simulink library "tp333079"  (Simulink 5.0)
values from neighbouring files (symbols this model uses):
  b = 1    [main_flock3.m]    (also in main_flock4.m; params_flocking_ros.m)
undefined symbols (not defined in the file or in its folder): AC, AlphaBnd, BetaBnd, CDda, CDde, CDdf, CDdr, CDM, CDmin, CGempty, CGgross, CL0, CLa, CLalphadot, Clbeta, Clda, CLde, CLdf, Cldr, CLM, CLmind, Clp, CLq, Clr, Cm0, Cma, Cmalphadot, Cmde, Cmdf, CmM, Cmq, Cnbeta, Cnda, Cndr, Cnp, Cnr, CP, CT, CYbeta, CYda, CYdr, CYp, CYr, Displacement, dmy, Engine, EulerIni, FuelFlow, FuelIni, J, Jempty, Jeng, Jgross, Jprop, MAC, MAP, MAPLim, MassIni, MaxPower, mempty ... (+26)
libraries: aerosimlib x325, simulink3 x42
(part 6 of 11)

== system tp333079/Complete Aircraft/6-DOF Aircraft Model (Body-frame EOM)/Atmosphere ==
  note: Inputs
  note: Outputs
  MSL : Inport  Port=1  PortDimensions=1  SampleTime=-1  DataType=double
      settings: SignalType=auto
  AGL : Inport  Port=2  PortDimensions=1  SampleTime=-1  DataType=double
      settings: SignalType=auto
  Winds : Inport  Port=3  PortDimensions=[3 1]  SampleTime=-1  DataType=double
      settings: SignalType=auto
  VelB : Inport  Port=4  PortDimensions=[3 1]  SampleTime=-1  DataType=double
      settings: SignalType=auto
  VelW : Inport  Port=5  PortDimensions=[3 1]  SampleTime=-1  DataType=auto
      settings: SignalType=auto
  DCM : Inport  Port=6  PortDimensions=[3 3]  SampleTime=-1  DataType=double
      settings: SignalType=auto
  Background Wind : aerosimlib/Atmosphere/Background Wind
  Standard Atmosphere : aerosimlib/Atmosphere/Standard Atmosphere
  Sum : Sum  Inputs=|++  SaturateOnIntegerOverflow=on
  Turbulence : aerosimlib/Atmosphere/Turbulence  tsamp=tsamp
  Wind Shear : aerosimlib/Atmosphere/Wind Shear
  pstatic : Outport  Port=1
  OAT : Outport  Port=2
  rho : Outport  Port=3
  a : Outport  Port=4
  WindVel : Outport  Port=5
  WindRates : Outport  Port=6
  wires:
  MSL/1 -> Standard Atmosphere/1
  Winds/1 -> Background Wind/1
  DCM/1 -> Background Wind/2
  Background Wind/1 -> Turbulence/3, Sum/2
  AGL/1 -> Turbulence/2
  VelW/1 -> Turbulence/1
  Background Wind/2 -> Wind Shear/1
  Turbulence/1 -> Sum/1
  Turbulence/2 -> Wind Shear/2
  VelB/1 -> Wind Shear/3
  Wind Shear/1 -> WindRates/1
  Standard Atmosphere/1 -> pstatic/1
  Standard Atmosphere/2 -> OAT/1
  Standard Atmosphere/3 -> rho/1
  Standard Atmosphere/4 -> a/1
  Sum/1 -> WindVel/1

== system tp333079/Complete Aircraft/6-DOF Aircraft Model (Body-frame EOM)/Earth ==
  note: Inputs
  note: Outputs
  Position : Inport  Port=1  PortDimensions=[3 1]  SampleTime=-1  DataType=double
      settings: SignalType=auto
  DCM : Inport  Port=2  PortDimensions=[3 3]  SampleTime=-1  DataType=double
      settings: SignalType=auto
  Demux : Demux  Outputs=2  BusSelectionMode=off
  ECEF Position : aerosimlib/Transformations/ECEF Position
  EGM-96 : aerosimlib/Earth/EGM-96
  Ground Alt : Constant  Value=GndAlt
  Ground Detection : aerosimlib/Earth/Ground Detection
  Mux3 : Mux  Inputs=2
  WGS-84 : aerosimlib/Earth/WGS-84
  WMM-2000 : aerosimlib/Earth/WMM-2000  wmmfile=wmmfile  simdate=dmy
  MSL : Outport  Port=1
  AGL : Outport  Port=2
  AConGnd : Outport  Port=3
  Rearth : Outport  Port=4
  Requiv : Outport  Port=5
  Gravity : Outport  Port=6
  MagField : Outport  Port=7
  ECEF : Outport  Port=8
  wires:
  Position/1 -> WGS-84/1, EGM-96/1, WMM-2000/1, ECEF Position/1
  DCM/1 -> WMM-2000/2
  Ground Alt/1 -> Ground Detection/2
  EGM-96/1 -> Ground Detection/1, MSL/1
  WGS-84/1 -> Mux3/1
  WGS-84/2 -> Mux3/2
  Ground Detection/2 -> AGL/1
  Ground Detection/1 -> AConGnd/1
  Mux3/1 -> Rearth/1, Demux/1
  WGS-84/3 -> Requiv/1
  WGS-84/4 -> Gravity/1
  WMM-2000/1 -> MagField/1
  Demux/1 -> ECEF Position/2
  Demux/2 -> ECEF Position/3
  ECEF Position/1 -> ECEF/1

== system tp333079/Complete Aircraft/6-DOF Aircraft Model (Body-frame EOM)/Equations of Motion ==
  note: Outputs
  note: Inputs
  Accel : Inport  Port=1  PortDimensions=[3 1]  SampleTime=-1  DataType=auto
      settings: SignalType=auto
  Moment : Inport  Port=2  PortDimensions=[3 1]  SampleTime=-1  DataType=auto
      settings: SignalType=auto
  Inertia : Inport  Port=3  PortDimensions=[4 1]  SampleTime=-1  DataType=auto
      settings: SignalType=auto
  Rearth : Inport  Port=4  PortDimensions=[2 1]  SampleTime=-1  DataType=auto
      settings: SignalType=auto
  Gravity : Inport  Port=5  PortDimensions=1  SampleTime=-1  DataType=auto
      settings: SignalType=auto
  AConGnd : Inport  Port=6  PortDimensions=1  SampleTime=-1  DataType=auto
      settings: SignalType=auto
  RST : Inport  Port=7  PortDimensions=1  SampleTime=-1  DataType=auto
      settings: SignalType=auto
  Body-Inertial DCM From Quaternions : aerosimlib/Transformations/Body-Inertial DCM From Quaternions
  Demux : Demux  Outputs=2  BusSelectionMode=off
  Euler Angles From Quaternions : aerosimlib/Transformations/Euler Angles From Quaternions
  Forces : aerosimlib/Equations of Motion/Body-Frame EOM/Forces  VelocitiesIni=VelocitiesIni
  Kinematics (Quaternions) : aerosimlib/Equations of Motion/Body-Frame EOM/Kinematics (Quaternions)  QuaternionsIni=QuaternionsIni
  Moments : aerosimlib/Equations of Motion/Body-Frame EOM/Moments  RatesIni=RatesIni
  Navigation : aerosimlib/Equations of Motion/Body-Frame EOM/Navigation  PositionIni=PositionIni
  VelB : Outport  Port=1
  Rates : Outport  Port=2
  Quaternions : Outport  Port=3
  Position : Outport  Port=4
  Groundspeed : Outport  Port=5
  DCM : Outport  Port=6
  Euler : Outport  Port=7
  Ang Acc : Outport  Port=8
  wires:
  Euler Angles From Quaternions/1 -> Euler/1
  Body-Inertial DCM From Quaternions/1 -> DCM/1, Forces/4, Navigation/2
  Rearth/1 -> Demux/1
  Demux/1 -> Navigation/3
  Demux/2 -> Navigation/4
  Accel/1 -> Forces/2
  Moment/1 -> Moments/2
  Inertia/1 -> Moments/1
  Gravity/1 -> Forces/3
  AConGnd/1 -> Navigation/5
  Forces/1 -> VelB/1, Navigation/1
  Kinematics (Quaternions)/1 -> Quaternions/1, Euler Angles From Quaternions/1, Body-Inertial DCM From Quaternions/1
  Moments/1 -> Forces/1, Kinematics (Quaternions)/1, Rates/1
  RST/1 -> Forces/5, Moments/3, Navigation/6, Kinematics (Quaternions)/2
  Moments/2 -> Ang Acc/1
  Navigation/1 -> Position/1
  Navigation/2 -> Groundspeed/1

== system tp333079/Complete Aircraft/6-DOF Aircraft Model (Geodetic-frame EOM)/Aerodynamics ==
  note: Aerodynamic Loads
  note: Aerodynamic Coefficients
  note: Aerodynamic Parameters
  note: Outputs
  note: Inputs
  VelB : Inport  Port=1  PortDimensions=[3 1]  SampleTime=-1  DataType=auto
      settings: SignalType=auto
  WindB : Inport  Port=2  PortDimensions=[3 1]  SampleTime=-1  DataType=auto
      settings: SignalType=auto
  Rates : Inport  Port=3  PortDimensions=[3 1]  SampleTime=-1  DataType=auto
      settings: SignalType=auto
  WindRates : Inport  Port=4  PortDimensions=[3 1]  SampleTime=-1  DataType=auto
      settings: SignalType=auto
  AeroCon : Inport  Port=5  PortDimensions=[4 1]  SampleTime=-1  DataType=auto
      settings: SignalType=auto
  rho : Inport  Port=6  PortDimensions=1  SampleTime=-1  DataType=auto
      settings: SignalType=auto
  a : Inport  Port=7  PortDimensions=1  SampleTime=-1  DataType=auto
      settings: SignalType=auto
  Aerodynamic Force : aerosimlib/Aerodynamics/Aerodynamic Force  S=S
  Aerodynamic Moment : aerosimlib/Aerodynamics/Aerodynamic Moment  c=MAC  b=b  S=S
  Drag Coefficient : aerosimlib/Aerodynamics/Drag Coefficient  CL0=CLmind  CD0=CDmin  CDdf=CDdf  CDde=CDde  CDda=CDda  CDdr=CDdr  CDM=CDM  e=osw  b=b  S=S
  Dynamic Pressure : aerosimlib/Aerodynamics/Dynamic Pressure
  Lift Coefficient : aerosimlib/Aerodynamics/Lift Coefficient  CL0=CL0  CLalpha=CLa  CLdf=CLdf  CLde=CLde  CLalphadot=CLalphadot  CLq=CLq  CLM=CLM  c=MAC
  Mux : Mux  Inputs=6
  Pitch Moment Coefficient : aerosimlib/Aerodynamics/Pitch Moment Coefficient  Cm0=Cm0  Cma=Cma  Cmdf=Cmdf  Cmde=Cmde  Cmalphadot=Cmalphadot  Cmq=Cmq  CmM=CmM  c=MAC
  Roll Moment Coefficient : aerosimlib/Aerodynamics/Roll Moment Coefficient  Clbeta=Clbeta  Clda=Clda  Cldr=Cldr  Clp=Clp  Clr=Clr  b=b
  Side Force Coefficient : aerosimlib/Aerodynamics/Side Force Coefficient  CYbeta=CYbeta  CYda=CYda  CYdr=CYdr  CYp=CYp  CYr=CYr  b=b
  Sum : Sum  Inputs=|+-  SaturateOnIntegerOverflow=on
  Wind-axes Velocities : aerosimlib/Aerodynamics/Wind-axes Velocities  Vabnd=VaBnd  betabnd=BetaBnd  alphabnd=AlphaBnd
  Yaw Moment Coefficient : aerosimlib/Aerodynamics/Yaw Moment Coefficient  Cnbeta=Cnbeta  Cnda=Cnda  Cndr=Cndr  Cnp=Cnp  Cnr=Cnr  b=b
  Faero : Outport  Port=1
  Maero : Outport  Port=2
  AeroCoeff : Outport  Port=3
  VelW : Outport  Port=4
  Mach : Outport  Port=5
  pdyn : Outport  Port=6
  wires:
  VelB/1 -> Wind-axes Velocities/1
  WindB/1 -> Wind-axes Velocities/2
  a/1 -> Wind-axes Velocities/3
  Wind-axes Velocities/1 -> Lift Coefficient/1, Dynamic Pressure/1, Drag Coefficient/1, Side Force Coefficient/1, Pitch Moment Coefficient/1, Roll Moment Coefficient/1, Yaw Moment Coefficient/1, Aerodynamic Force/5, VelW/1
  rho/1 -> Dynamic Pressure/2
  AeroCon/1 -> Lift Coefficient/2, Drag Coefficient/2, Side Force Coefficient/2, Pitch Moment Coefficient/2, Roll Moment Coefficient/2, Yaw Moment Coefficient/2
  Wind-axes Velocities/2 -> Lift Coefficient/3, Pitch Moment Coefficient/3
  Wind-axes Velocities/3 -> Drag Coefficient/4, Pitch Moment Coefficient/5, Lift Coefficient/5, Mach/1
  Lift Coefficient/1 -> Aerodynamic Force/3, Drag Coefficient/3, Mux/3
  Drag Coefficient/1 -> Aerodynamic Force/1, Mux/1
  Side Force Coefficient/1 -> Aerodynamic Force/2, Mux/2
  Dynamic Pressure/1 -> Aerodynamic Force/4, Aerodynamic Moment/4, pdyn/1
  Roll Moment Coefficient/1 -> Aerodynamic Moment/1, Mux/4
  Pitch Moment Coefficient/1 -> Aerodynamic Moment/2, Mux/5
  Yaw Moment Coefficient/1 -> Aerodynamic Moment/3, Mux/6
  Aerodynamic Force/1 -> Faero/1
  Aerodynamic Moment/1 -> Maero/1
  Mux/1 -> AeroCoeff/1
  Rates/1 -> Sum/1
  WindRates/1 -> Sum/2
  Sum/1 -> Lift Coefficient/4, Side Force Coefficient/3, Pitch Moment Coefficient/4, Yaw Moment Coefficient/3, Roll Moment Coefficient/3

== system tp333079/Complete Aircraft/6-DOF Aircraft Model (Geodetic-frame EOM)/Atmosphere ==
  note: Inputs
  note: Outputs
  MSL : Inport  Port=1  PortDimensions=1  SampleTime=-1  DataType=double
      settings: SignalType=auto
  AGL : Inport  Port=2  PortDimensions=1  SampleTime=-1  DataType=double
      settings: SignalType=auto
  Winds : Inport  Port=3  PortDimensions=[3 1]  SampleTime=-1  DataType=double
      settings: SignalType=auto
  VelB : Inport  Port=4  PortDimensions=[3 1]  SampleTime=-1  DataType=double
      settings: SignalType=auto
  VelW : Inport  Port=5  PortDimensions=[3 1]  SampleTime=-1  DataType=auto
      settings: SignalType=auto
  DCM : Inport  Port=6  PortDimensions=[3 3]  SampleTime=-1  DataType=double
      settings: SignalType=auto
  Background Wind : aerosimlib/Atmosphere/Background Wind
  Standard Atmosphere : aerosimlib/Atmosphere/Standard Atmosphere
  Sum : Sum  Inputs=|++  SaturateOnIntegerOverflow=on
  Turbulence : aerosimlib/Atmosphere/Turbulence  tsamp=tsamp
  Wind Shear : aerosimlib/Atmosphere/Wind Shear
  pstatic : Outport  Port=1
  OAT : Outport  Port=2
  rho : Outport  Port=3
  a : Outport  Port=4
  WindVel : Outport  Port=5
  WindRates : Outport  Port=6
  wires:
  MSL/1 -> Standard Atmosphere/1
  Winds/1 -> Background Wind/1
  DCM/1 -> Background Wind/2
  Background Wind/1 -> Turbulence/3, Sum/2
  AGL/1 -> Turbulence/2
  VelW/1 -> Turbulence/1
  Background Wind/2 -> Wind Shear/1
  Turbulence/1 -> Sum/1
  Turbulence/2 -> Wind Shear/2
  VelB/1 -> Wind Shear/3
  Wind Shear/1 -> WindRates/1
  Standard Atmosphere/1 -> pstatic/1
  Standard Atmosphere/2 -> OAT/1
  Standard Atmosphere/3 -> rho/1
  Standard Atmosphere/4 -> a/1
  Sum/1 -> WindVel/1

== system tp333079/Complete Aircraft/6-DOF Aircraft Model (Geodetic-frame EOM)/Earth ==
  note: Inputs
  note: Outputs
  Position : Inport  Port=1  PortDimensions=[3 1]  SampleTime=-1  DataType=double
      settings: SignalType=auto
  DCM : Inport  Port=2  PortDimensions=[3 3]  SampleTime=-1  DataType=double
      settings: SignalType=auto
  Demux : Demux  Outputs=2  BusSelectionMode=off
  ECEF Position : aerosimlib/Transformations/ECEF Position
  EGM-96 : aerosimlib/Earth/EGM-96
  Ground Alt : Constant  Value=GndAlt
  Ground Detection : aerosimlib/Earth/Ground Detection
  Mux3 : Mux  Inputs=2
  WGS-84 : aerosimlib/Earth/WGS-84
  WMM-2000 : aerosimlib/Earth/WMM-2000  wmmfile=wmmfile  simdate=dmy
  MSL : Outport  Port=1
  AGL : Outport  Port=2
  AConGnd : Outport  Port=3
  Rearth : Outport  Port=4
  Requiv : Outport  Port=5
  Gravity : Outport  Port=6
  MagField : Outport  Port=7
  ECEF : Outport  Port=8
  wires:
  Position/1 -> WGS-84/1, EGM-96/1, WMM-2000/1, ECEF Position/1
  DCM/1 -> WMM-2000/2
  Ground Alt/1 -> Ground Detection/2
  EGM-96/1 -> Ground Detection/1, MSL/1
  WGS-84/1 -> Mux3/1
  WGS-84/2 -> Mux3/2
  Ground Detection/2 -> AGL/1
  Ground Detection/1 -> AConGnd/1
  Mux3/1 -> Rearth/1, Demux/1
  WGS-84/3 -> Requiv/1
  WGS-84/4 -> Gravity/1
  WMM-2000/1 -> MagField/1
  Demux/1 -> ECEF Position/2
  Demux/2 -> ECEF Position/3
  ECEF Position/1 -> ECEF/1

== system tp333079/Complete Aircraft/6-DOF Aircraft Model (Geodetic-frame EOM)/Equations of Motion ==
  note: Inputs
  note: Outputs
  Accel : Inport  Port=1  PortDimensions=[3 1]  SampleTime=-1  DataType=auto
      settings: SignalType=auto
  Moment : Inport  Port=2  PortDimensions=[3 1]  SampleTime=-1  DataType=auto
      settings: SignalType=auto
  Inertia : Inport  Port=3  PortDimensions=[4 1]  SampleTime=-1  DataType=auto
      settings: SignalType=auto
  Rearth : Inport  Port=4  PortDimensions=[2 1]  SampleTime=-1  DataType=auto
      settings: SignalType=auto
  Gravity : Inport  Port=5  PortDimensions=1  SampleTime=-1  DataType=auto
      settings: SignalType=auto
  AConGnd : Inport  Port=6  PortDimensions=1  SampleTime=-1  DataType=auto
      settings: SignalType=auto
  RST : Inport  Port=7  PortDimensions=1  SampleTime=-1  DataType=auto
      settings: SignalType=auto
  Angular Rate : aerosimlib/Equations of Motion/Geodetic-Frame EOM/Angular Rate  RatesIni=RatesIni
  Attitude : aerosimlib/Equations of Motion/Body-Frame EOM/Kinematics (Quaternions)  QuaternionsIni=QuaternionsIni
  Body-Inertial DCM : aerosimlib/Transformations/Body-Inertial DCM From Quaternions
  Demux : Demux  Outputs=2  BusSelectionMode=off
  Euler Angles : aerosimlib/Transformations/Euler Angles From Quaternions
  Position : aerosimlib/Equations of Motion/Geodetic-Frame EOM/Position  PositionIni=PositionIni
  Product : Product  Inputs=2  Multiplication=Matrix(*)  SaturateOnIntegerOverflow=on
  Velocity : aerosimlib/Equations of Motion/Geodetic-Frame EOM/Velocity  VelocitiesIni=VelocitiesIni
  VelB : Outport  Port=1
  VelNED : Outport  Port=2
  Rates : Outport  Port=3
  Quaternions : Outport  Port=4
  Pos : Outport  Port=5
  Groundspeed : Outport  Port=6
  DCM : Outport  Port=7
  Euler : Outport  Port=8
  Ang Acc : Outport  Port=9
  wires:
  Attitude/1 -> Body-Inertial DCM/1, Euler Angles/1, Quaternions/1
  Position/1 -> Velocity/1, Angular Rate/3, Pos/1
  Position/2 -> Velocity/2, Angular Rate/4
  Velocity/1 -> Product/2, Position/1, Groundspeed/1, VelNED/1
  Demux/1 -> Position/2
  Demux/2 -> Position/3
  Rearth/1 -> Demux/1
  Gravity/1 -> Velocity/5
  RST/1 -> Velocity/6, Position/5, Attitude/2, Angular Rate/6
  Angular Rate/1 -> Attitude/1, Rates/1
  Moment/1 -> Angular Rate/2
  Inertia/1 -> Angular Rate/1
  Body-Inertial DCM/1 -> Angular Rate/5, Velocity/4, Product/1, DCM/1
  AConGnd/1 -> Position/4
  Accel/1 -> Velocity/3
  Product/1 -> VelB/1
  Angular Rate/2 -> Ang Acc/1
  Euler Angles/1 -> Euler/1

== system tp333079/Complete Aircraft/6-DOF Aircraft Model (Geodetic-frame EOM) No magnetic field/Aerodynamics ==
  note: Inputs
  note: Outputs
  note: Aerodynamic Parameters
  note: Aerodynamic Coefficients
  note: Aerodynamic Loads
  VelB : Inport  Port=1  PortDimensions=[3 1]  SampleTime=-1  DataType=auto
      settings: SignalType=auto
  WindB : Inport  Port=2  PortDimensions=[3 1]  SampleTime=-1  DataType=auto
      settings: SignalType=auto
  Rates : Inport  Port=3  PortDimensions=[3 1]  SampleTime=-1  DataType=auto
      settings: SignalType=auto
  WindRates : Inport  Port=4  PortDimensions=[3 1]  SampleTime=-1  DataType=auto
      settings: SignalType=auto
  AeroCon : Inport  Port=5  PortDimensions=[4 1]  SampleTime=-1  DataType=auto
      settings: SignalType=auto
  rho : Inport  Port=6  PortDimensions=1  SampleTime=-1  DataType=auto
      settings: SignalType=auto
  a : Inport  Port=7  PortDimensions=1  SampleTime=-1  DataType=auto
      settings: SignalType=auto
  Aerodynamic Force : aerosimlib/Aerodynamics/Aerodynamic Force  S=S
  Aerodynamic Moment : aerosimlib/Aerodynamics/Aerodynamic Moment  c=MAC  b=b  S=S
  Drag Coefficient : aerosimlib/Aerodynamics/Drag Coefficient  CL0=CLmind  CD0=CDmin  CDdf=CDdf  CDde=CDde  CDda=CDda  CDdr=CDdr  CDM=CDM  e=osw  b=b  S=S
  Dynamic Pressure : aerosimlib/Aerodynamics/Dynamic Pressure
  Lift Coefficient : aerosimlib/Aerodynamics/Lift Coefficient  CL0=CL0  CLalpha=CLa  CLdf=CLdf  CLde=CLde  CLalphadot=CLalphadot  CLq=CLq  CLM=CLM  c=MAC
  Mux : Mux  Inputs=6
  Pitch Moment Coefficient : aerosimlib/Aerodynamics/Pitch Moment Coefficient  Cm0=Cm0  Cma=Cma  Cmdf=Cmdf  Cmde=Cmde  Cmalphadot=Cmalphadot  Cmq=Cmq  CmM=CmM  c=MAC
  Roll Moment Coefficient : aerosimlib/Aerodynamics/Roll Moment Coefficient  Clbeta=Clbeta  Clda=Clda  Cldr=Cldr  Clp=Clp  Clr=Clr  b=b
  Side Force Coefficient : aerosimlib/Aerodynamics/Side Force Coefficient  CYbeta=CYbeta  CYda=CYda  CYdr=CYdr  CYp=CYp  CYr=CYr  b=b
  Sum : Sum  Inputs=|+-  SaturateOnIntegerOverflow=on
  Wind-axes Velocities : aerosimlib/Aerodynamics/Wind-axes Velocities  Vabnd=VaBnd  betabnd=BetaBnd  alphabnd=AlphaBnd
  Yaw Moment Coefficient : aerosimlib/Aerodynamics/Yaw Moment Coefficient  Cnbeta=Cnbeta  Cnda=Cnda  Cndr=Cndr  Cnp=Cnp  Cnr=Cnr  b=b
  Faero : Outport  Port=1
  Maero : Outport  Port=2
  AeroCoeff : Outport  Port=3
  VelW : Outport  Port=4
  Mach : Outport  Port=5
  pdyn : Outport  Port=6
  wires:
  Sum/1 -> Roll Moment Coefficient/3, Yaw Moment Coefficient/3, Pitch Moment Coefficient/4, Side Force Coefficient/3, Lift Coefficient/4
  WindRates/1 -> Sum/2
  Rates/1 -> Sum/1
  Mux/1 -> AeroCoeff/1
  Aerodynamic Moment/1 -> Maero/1
  Aerodynamic Force/1 -> Faero/1
  Yaw Moment Coefficient/1 -> Mux/6, Aerodynamic Moment/3
  Pitch Moment Coefficient/1 -> Mux/5, Aerodynamic Moment/2
  Roll Moment Coefficient/1 -> Mux/4, Aerodynamic Moment/1
  Dynamic Pressure/1 -> pdyn/1, Aerodynamic Moment/4, Aerodynamic Force/4
  Side Force Coefficient/1 -> Mux/2, Aerodynamic Force/2
  Drag Coefficient/1 -> Mux/1, Aerodynamic Force/1
  Lift Coefficient/1 -> Mux/3, Drag Coefficient/3, Aerodynamic Force/3
  Wind-axes Velocities/3 -> Mach/1, Lift Coefficient/5, Pitch Moment Coefficient/5, Drag Coefficient/4
  Wind-axes Velocities/2 -> Pitch Moment Coefficient/3, Lift Coefficient/3
  AeroCon/1 -> Yaw Moment Coefficient/2, Roll Moment Coefficient/2, Pitch Moment Coefficient/2, Side Force Coefficient/2, Drag Coefficient/2, Lift Coefficient/2
  rho/1 -> Dynamic Pressure/2
  Wind-axes Velocities/1 -> VelW/1, Aerodynamic Force/5, Yaw Moment Coefficient/1, Roll Moment Coefficient/1, Pitch Moment Coefficient/1, Side Force Coefficient/1, Drag Coefficient/1, Dynamic Pressure/1, Lift Coefficient/1
  a/1 -> Wind-axes Velocities/3
  WindB/1 -> Wind-axes Velocities/2
  VelB/1 -> Wind-axes Velocities/1

== system tp333079/Complete Aircraft/6-DOF Aircraft Model (Geodetic-frame EOM) No magnetic field/Atmosphere ==
  note: Outputs
  note: Inputs
  MSL : Inport  Port=1  PortDimensions=1  SampleTime=-1  DataType=double
      settings: SignalType=auto
  AGL : Inport  Port=2  PortDimensions=1  SampleTime=-1  DataType=double
      settings: SignalType=auto
  Winds : Inport  Port=3  PortDimensions=[3 1]  SampleTime=-1  DataType=double
      settings: SignalType=auto
  VelB : Inport  Port=4  PortDimensions=[3 1]  SampleTime=-1  DataType=double
      settings: SignalType=auto
  VelW : Inport  Port=5  PortDimensions=[3 1]  SampleTime=-1  DataType=auto
      settings: SignalType=auto
  DCM : Inport  Port=6  PortDimensions=[3 3]  SampleTime=-1  DataType=double
      settings: SignalType=auto
  Background Wind : aerosimlib/Atmosphere/Background Wind
  Standard Atmosphere : aerosimlib/Atmosphere/Standard Atmosphere
  Sum : Sum  Inputs=|++  SaturateOnIntegerOverflow=on
  Turbulence : aerosimlib/Atmosphere/Turbulence  tsamp=tsamp
  Wind Shear : aerosimlib/Atmosphere/Wind Shear
  pstatic : Outport  Port=1
  OAT : Outport  Port=2
  rho : Outport  Port=3
  a : Outport  Port=4
  WindVel : Outport  Port=5
  WindRates : Outport  Port=6
  wires:
  Sum/1 -> WindVel/1
  Standard Atmosphere/4 -> a/1
  Standard Atmosphere/3 -> rho/1
  Standard Atmosphere/2 -> OAT/1
  Standard Atmosphere/1 -> pstatic/1
  Wind Shear/1 -> WindRates/1
  VelB/1 -> Wind Shear/3
  Turbulence/2 -> Wind Shear/2
  Turbulence/1 -> Sum/1
  Background Wind/2 -> Wind Shear/1
  VelW/1 -> Turbulence/1
  AGL/1 -> Turbulence/2
  Background Wind/1 -> Sum/2, Turbulence/3
  DCM/1 -> Background Wind/2
  Winds/1 -> Background Wind/1
  MSL/1 -> Standard Atmosphere/1

== system tp333079/Complete Aircraft/6-DOF Aircraft Model (Geodetic-frame EOM) No magnetic field/Earth ==
  note: Outputs
  note: Inputs
  Position : Inport  Port=1  PortDimensions=[3 1]  SampleTime=-1  DataType=double
      settings: SignalType=auto
  Demux : Demux  Outputs=2  BusSelectionMode=off
  ECEF Position : aerosimlib/Transformations/ECEF Position
  EGM-96 : aerosimlib/Earth/EGM-96
  Ground Alt : Constant  Value=GndAlt
  Ground Detection : aerosimlib/Earth/Ground Detection
  Mux3 : Mux  Inputs=2
  WGS-84 : aerosimlib/Earth/WGS-84
  MSL : Outport  Port=1
  AGL : Outport  Port=2
  AConGnd : Outport  Port=3
  Rearth : Outport  Port=4
  Requiv : Outport  Port=5
  Gravity : Outport  Port=6
  ECEF : Outport  Port=7
  wires:
  ECEF Position/1 -> ECEF/1
  Demux/2 -> ECEF Position/3
  Demux/1 -> ECEF Position/2
  WGS-84/4 -> Gravity/1
  WGS-84/3 -> Requiv/1
  Mux3/1 -> Demux/1, Rearth/1
  Ground Detection/1 -> AConGnd/1
  Ground Detection/2 -> AGL/1
  WGS-84/2 -> Mux3/2
  WGS-84/1 -> Mux3/1
  EGM-96/1 -> MSL/1, Ground Detection/1
  Ground Alt/1 -> Ground Detection/2
  Position/1 -> EGM-96/1, ECEF Position/1, WGS-84/1

== system tp333079/Complete Aircraft/6-DOF Aircraft Model (Geodetic-frame EOM) No magnetic field/Equations of Motion ==
  note: Outputs
  note: Inputs
  Accel : Inport  Port=1  PortDimensions=[3 1]  SampleTime=-1  DataType=auto
      settings: SignalType=auto
  Moment : Inport  Port=2  PortDimensions=[3 1]  SampleTime=-1  DataType=auto
      settings: SignalType=auto
  Inertia : Inport  Port=3  PortDimensions=[4 1]  SampleTime=-1  DataType=auto
      settings: SignalType=auto
  Rearth : Inport  Port=4  PortDimensions=[2 1]  SampleTime=-1  DataType=auto
      settings: SignalType=auto
  Gravity : Inport  Port=5  PortDimensions=1  SampleTime=-1  DataType=auto
      settings: SignalType=auto
  AConGnd : Inport  Port=6  PortDimensions=1  SampleTime=-1  DataType=auto
      settings: SignalType=auto
  RST : Inport  Port=7  PortDimensions=1  SampleTime=-1  DataType=auto
      settings: SignalType=auto
  Angular Rate : aerosimlib/Equations of Motion/Geodetic-Frame EOM/Angular Rate  RatesIni=RatesIni
  Attitude : aerosimlib/Equations of Motion/Body-Frame EOM/Kinematics (Quaternions)  QuaternionsIni=QuaternionsIni
  Body-Inertial DCM : aerosimlib/Transformations/Body-Inertial DCM From Quaternions
  Demux : Demux  Outputs=2  BusSelectionMode=off
  Euler Angles : aerosimlib/Transformations/Euler Angles From Quaternions
  Position : aerosimlib/Equations of Motion/Geodetic-Frame EOM/Position  PositionIni=PositionIni
  Product : Product  Inputs=2  Multiplication=Matrix(*)  SaturateOnIntegerOverflow=on
  Velocity : aerosimlib/Equations of Motion/Geodetic-Frame EOM/Velocity  VelocitiesIni=VelocitiesIni
  VelB : Outport  Port=1
  VelNED : Outport  Port=2
  Rates : Outport  Port=3
  Quaternions : Outport  Port=4
  Pos : Outport  Port=5
  Groundspeed : Outport  Port=6
  DCM : Outport  Port=7
  Euler : Outport  Port=8
  Ang Acc : Outport  Port=9
  wires:
  Euler Angles/1 -> Euler/1
  Angular Rate/2 -> Ang Acc/1
  Product/1 -> VelB/1
  Accel/1 -> Velocity/3
  AConGnd/1 -> Position/4
  Body-Inertial DCM/1 -> DCM/1, Product/1, Velocity/4, Angular Rate/5
  Inertia/1 -> Angular Rate/1
  Moment/1 -> Angular Rate/2
  Angular Rate/1 -> Rates/1, Attitude/1
  RST/1 -> Angular Rate/6, Attitude/2, Position/5, Velocity/6
  Gravity/1 -> Velocity/5
  Rearth/1 -> Demux/1
  Demux/2 -> Position/3
  Demux/1 -> Position/2
  Velocity/1 -> VelNED/1, Groundspeed/1, Position/1, Product/2
  Position/2 -> Angular Rate/4, Velocity/2
  Position/1 -> Pos/1, Angular Rate/3, Velocity/1
  Attitude/1 -> Quaternions/1, Euler Angles/1, Body-Inertial DCM/1

== system tp333079/Complete Aircraft/Glider Model/Equations of Motion ==
  note: Inputs
  note: Outputs
  Accel : Inport  Port=1  PortDimensions=[3 1]  SampleTime=-1  DataType=auto
      settings: SignalType=auto
  Moment : Inport  Port=2  PortDimensions=[3 1]  SampleTime=-1  DataType=auto
      settings: SignalType=auto
  Inertia : Inport  Port=3  PortDimensions=[4 1]  SampleTime=-1  DataType=auto
      settings: SignalType=auto
  Rearth : Inport  Port=4  PortDimensions=[2 1]  SampleTime=-1  DataType=auto
      settings: SignalType=auto
  Gravity : Inport  Port=5  PortDimensions=1  SampleTime=-1  DataType=auto
      settings: SignalType=auto
  AConGnd : Inport  Port=6  PortDimensions=1  SampleTime=-1  DataType=auto
      settings: SignalType=auto
  RST : Inport  Port=7  PortDimensions=1  SampleTime=-1  DataType=auto
      settings: SignalType=auto
  Body-Inertial DCM From Quaternions : aerosimlib/Transformations/Body-Inertial DCM From Quaternions
  Demux : Demux  Outputs=2  BusSelectionMode=off
  Euler Angles From Quaternions : aerosimlib/Transformations/Euler Angles From Quaternions
  Forces : aerosimlib/Equations of Motion/Body-Frame EOM/Forces  VelocitiesIni=VelocitiesIni
  Kinematics (Quaternions) : aerosimlib/Equations of Motion/Body-Frame EOM/Kinematics (Quaternions)  QuaternionsIni=QuaternionsIni
  Moments : aerosimlib/Equations of Motion/Body-Frame EOM/Moments  RatesIni=RatesIni
  Navigation : aerosimlib/Equations of Motion/Body-Frame EOM/Navigation  PositionIni=PositionIni
  VelB : Outport  Port=1
  Rates : Outport  Port=2
  Quaternions : Outport  Port=3
  Position : Outport  Port=4
  Groundspeed : Outport  Port=5
  DCM : Outport  Port=6
  Euler : Outport  Port=7
  Ang Acc : Outport  Port=8
  wires:
  Navigation/2 -> Groundspeed/1
  Navigation/1 -> Position/1
  Moments/2 -> Ang Acc/1
  RST/1 -> Kinematics (Quaternions)/2, Navigation/6, Moments/3, Forces/5
  Moments/1 -> Rates/1, Kinematics (Quaternions)/1, Forces/1
  Kinematics (Quaternions)/1 -> Body-Inertial DCM From Quaternions/1, Euler Angles From Quaternions/1, Quaternions/1
  Forces/1 -> Navigation/1, VelB/1
  AConGnd/1 -> Navigation/5
  Gravity/1 -> Forces/3
  Inertia/1 -> Moments/1
  Moment/1 -> Moments/2
  Accel/1 -> Forces/2
  Demux/2 -> Navigation/4
  Demux/1 -> Navigation/3
  Rearth/1 -> Demux/1
  Body-Inertial DCM From Quaternions/1 -> Navigation/2, Forces/4, DCM/1
  Euler Angles From Quaternions/1 -> Euler/1

== system tp333079/Complete Aircraft/Simple Aircraft Model/Equations of Motion ==
  note: Inputs
  note: Outputs
  Accel : Inport  Port=1  PortDimensions=[3 1]  SampleTime=-1  DataType=auto
      settings: SignalType=auto
  Moment : Inport  Port=2  PortDimensions=[3 1]  SampleTime=-1  DataType=auto
      settings: SignalType=auto
  Inertia : Inport  Port=3  PortDimensions=[4 1]  SampleTime=-1  DataType=auto
      settings: SignalType=auto
  Rearth : Inport  Port=4  PortDimensions=[2 1]  SampleTime=-1  DataType=auto
      settings: SignalType=auto
  Gravity : Inport  Port=5  PortDimensions=1  SampleTime=-1  DataType=auto
      settings: SignalType=auto
  AConGnd : Inport  Port=6  PortDimensions=1  SampleTime=-1  DataType=auto
      settings: SignalType=auto
  RST : Inport  Port=7  PortDimensions=1  SampleTime=-1  DataType=auto
      settings: SignalType=auto
  Body-Inertial DCM From Quaternions : aerosimlib/Transformations/Body-Inertial DCM From Quaternions
  Demux : Demux  Outputs=2  BusSelectionMode=off
  Euler Angles From Quaternions : aerosimlib/Transformations/Euler Angles From Quaternions
  Forces : aerosimlib/Equations of Motion/Body-Frame EOM/Forces  VelocitiesIni=VelocitiesIni
  Kinematics (Quaternions) : aerosimlib/Equations of Motion/Body-Frame EOM/Kinematics (Quaternions)  QuaternionsIni=QuaternionsIni
  Moments : aerosimlib/Equations of Motion/Body-Frame EOM/Moments  RatesIni=RatesIni
  Navigation : aerosimlib/Equations of Motion/Body-Frame EOM/Navigation  PositionIni=PositionIni
  VelB : Outport  Port=1
  Rates : Outport  Port=2
  Quaternions : Outport  Port=3
  Position : Outport  Port=4
  Groundspeed : Outport  Port=5
  DCM : Outport  Port=6
  Euler : Outport  Port=7
  Ang Acc : Outport  Port=8
  wires:
  Navigation/2 -> Groundspeed/1
  Navigation/1 -> Position/1
  Moments/2 -> Ang Acc/1
  RST/1 -> Kinematics (Quaternions)/2, Navigation/6, Moments/3, Forces/5
  Moments/1 -> Rates/1, Kinematics (Quaternions)/1, Forces/1
  Kinematics (Quaternions)/1 -> Body-Inertial DCM From Quaternions/1, Euler Angles From Quaternions/1, Quaternions/1
  Forces/1 -> Navigation/1, VelB/1
  AConGnd/1 -> Navigation/5
  Gravity/1 -> Forces/3
  Inertia/1 -> Moments/1
  Moment/1 -> Moments/2
  Accel/1 -> Forces/2
  Demux/2 -> Navigation/4
  Demux/1 -> Navigation/3
  Rearth/1 -> Demux/1
  Body-Inertial DCM From Quaternions/1 -> Navigation/2, Forces/4, DCM/1
  Euler Angles From Quaternions/1 -> Euler/1

== system tp333079/Earth/EGM-96/Longitude Bound 0-2pi ==
  In : Inport  Port=1  PortDimensions=-1  SampleTime=-1  DataType=auto
      settings: SignalType=auto
  2pi : Constant  Value=2*pi
  Math Function : Math  Operator=mod  OutputSignalType=auto
  Out : Outport  Port=1
  wires:
  Math Function/1 -> Out/1
  2pi/1 -> Math Function/2
  In/1 -> Math Function/1

== system tp333079/Earth/EGM-96/rad 2 deg ==
  In : Inport  Port=1  PortDimensions=-1  SampleTime=-1  DataType=auto
      settings: SignalType=auto
  Gain : Gain  Gain=180/pi  Multiplication=Element-wise(K.*u)  SaturateOnIntegerOverflow=on
  Out : Outport  Port=1
  wires:
  In/1 -> Gain/1
  Gain/1 -> Out/1

== system tp333079/Earth/EGM-96/rad 2 deg1 ==
  In : Inport  Port=1  PortDimensions=-1  SampleTime=-1  DataType=auto
      settings: SignalType=auto
  Gain : Gain  Gain=180/pi  Multiplication=Element-wise(K.*u)  SaturateOnIntegerOverflow=on
  Out : Outport  Port=1
  wires:
  Gain/1 -> Out/1
  In/1 -> Gain/1

== system tp333079/Equations of Motion/Body-Frame EOM/Forces ==
  note: Output
  note: Force equation
  note: Products
  note: Sources
  note: Gravity vector in body frame
  Rates : Inport  Port=1  PortDimensions=[3 1]  SampleTime=-1  DataType=auto
      settings: SignalType=auto
  Accel : Inport  Port=2  PortDimensions=[3 1]  SampleTime=-1  DataType=auto
      settings: SignalType=auto
  Gravity : Inport  Port=3  PortDimensions=1  SampleTime=-1  DataType=auto
      settings: SignalType=auto
  DCM : Inport  Port=4  PortDimensions=[3 3]  SampleTime=-1  DataType=auto
      settings: SignalType=auto
  RST : Inport  Port=5  PortDimensions=1  SampleTime=-1  DataType=auto
      settings: SignalType=auto
  Demux : Demux  Outputs=3  BusSelectionMode=off
  Demux2 : Demux  Outputs=3  BusSelectionMode=off
  Demux3 : Demux  Outputs=3  BusSelectionMode=off
  Mux : Mux  Inputs=3
  Mux1 : Mux  Inputs=3
  Product : Product  Inputs=2  Multiplication=Matrix(*)  SaturateOnIntegerOverflow=on
  Sum : Sum  Inputs=+-+  SaturateOnIntegerOverflow=on
  Sum1 : Sum  Inputs=-++  SaturateOnIntegerOverflow=on
  Sum2 : Sum  Inputs=+-+  SaturateOnIntegerOverflow=on
  Sum3 : Sum  Inputs=++  SaturateOnIntegerOverflow=on
  Velocity Integrator : Integrator  ExternalReset=rising  InitialConditionSource=internal  InitialCondition=VelocitiesIni  LimitOutput=off  UpperSaturationLimit=inf  LowerSaturationLimit=-inf  ShowSaturationPort=off  ShowStatePort=off  AbsoluteTolerance=auto
  Zero : Constant  Value=0
  pv : Product  Inputs=2  Multiplication=Element-wise(.*)  SaturateOnIntegerOverflow=on
  pw : Product  Inputs=2  Multiplication=Element-wise(.*)  SaturateOnIntegerOverflow=on
  qu : Product  Inputs=2  Multiplication=Element-wise(.*)  SaturateOnIntegerOverflow=on
  qw : Product  Inputs=2  Multiplication=Element-wise(.*)  SaturateOnIntegerOverflow=on
  ru : Product  Inputs=2  Multiplication=Element-wise(.*)  SaturateOnIntegerOverflow=on
  rv : Product  Inputs=2  Multiplication=Element-wise(.*)  SaturateOnIntegerOverflow=on
  Velocities : Outport  Port=1
  wires:
  Demux3/3 -> pw/2, qw/2
  Demux3/2 -> pv/2, rv/2
  Demux3/1 -> qu/2, ru/2
  Velocity Integrator/1 -> Velocities/1, Demux3/1
  RST/1 -> Velocity Integrator/2
  Mux/1 -> Velocity Integrator/1
  Sum2/1 -> Mux/3
  Sum1/1 -> Mux/2
  Sum/1 -> Mux/1
  pv/1 -> Sum2/2
  qu/1 -> Sum2/1
  pw/1 -> Sum1/2
  ru/1 -> Sum1/1
  Demux2/2 -> Sum1/3
  Demux2/3 -> Sum2/3
  Demux2/1 -> Sum/3
  Rates/1 -> Demux/1
  Demux/2 -> qw/1, qu/1
  Demux/3 -> ru/1, rv/1
  Demux/1 -> pw/1, pv/1
  rv/1 -> Sum/1
  qw/1 -> Sum/2
  DCM/1 -> Product/1
  Mux1/1 -> Product/2
  Gravity/1 -> Mux1/3
  Zero/1 -> Mux1/1, Mux1/2
  Sum3/1 -> Demux2/1
  Accel/1 -> Sum3/1
  Product/1 -> Sum3/2

== system tp333079/Equations of Motion/Body-Frame EOM/Kinematics (Euler) ==
  note: Sources
  note: Kinematic Equation
  note: Output
  Rates : Inport  Port=1  PortDimensions=[3 1]  SampleTime=-1  DataType=auto
      settings: SignalType=auto
  RST : Inport  Port=2  PortDimensions=1  SampleTime=-1  DataType=auto
      settings: SignalType=auto
  (qsin(phi)+rcos(phi))/cos(theta) : Product  Inputs=*/  Multiplication=Element-wise(.*)  SaturateOnIntegerOverflow=on
  2pi Bound : aerosimlib/Math/2pi Bound
  Demux : Demux  Outputs=3  BusSelectionMode=off
  Demux1 : Demux  Outputs=3  BusSelectionMode=off
  Demux2 : Demux  Outputs=3  BusSelectionMode=off
  Euler Angles Integrator : Integrator  ExternalReset=rising  InitialConditionSource=internal  InitialCondition=EulerIni  LimitOutput=off  UpperSaturationLimit=inf  LowerSaturationLimit=-inf  ShowSaturationPort=off  ShowStatePort=off  AbsoluteTolerance=auto
  Mux : Mux  Inputs=3
  Mux1 : Mux  Inputs=3
  Sum : Sum  Inputs=++  SaturateOnIntegerOverflow=on
  Sum1 : Sum  Inputs=+-  SaturateOnIntegerOverflow=on
  Sum2 : Sum  Inputs=++  SaturateOnIntegerOverflow=on
  Terminator : Terminator
  cos(phi) : Trigonometry  Operator=cos  OutputSignalType=auto
  cos(theta) : Trigonometry  Operator=cos  OutputSignalType=auto
  pi Bound : aerosimlib/Math/pi Bound
  pi Bound1 : aerosimlib/Math/pi Bound
  qcos(phi) : Product  Inputs=2  Multiplication=Element-wise(.*)  SaturateOnIntegerOverflow=on
  qsin(phi) : Product  Inputs=2  Multiplication=Element-wise(.*)  SaturateOnIntegerOverflow=on
  rcos(phi) : Product  Inputs=2  Multiplication=Element-wise(.*)  SaturateOnIntegerOverflow=on
  rsin(phi) : Product  Inputs=2  Multiplication=Element-wise(.*)  SaturateOnIntegerOverflow=on
  sin(phi) : Trigonometry  Operator=sin  OutputSignalType=auto
  tan(theta) : Trigonometry  Operator=tan  OutputSignalType=auto
  tan(theta)(qsin(phi)+rcos(phi)) : Product  Inputs=2  Multiplication=Element-wise(.*)  SaturateOnIntegerOverflow=on
  Euler : Outport  Port=1
  wires:
  Rates/1 -> Demux/1
  RST/1 -> Euler Angles Integrator/2
  Demux1/1 -> sin(phi)/1, cos(phi)/1
  Demux1/2 -> cos(theta)/1, tan(theta)/1
  Demux1/3 -> Terminator/1
  Demux/2 -> qsin(phi)/1, qcos(phi)/1
  Demux/3 -> rcos(phi)/1, rsin(phi)/1
  sin(phi)/1 -> qsin(phi)/2, rsin(phi)/2
  cos(phi)/1 -> rcos(phi)/2, qcos(phi)/2
  qsin(phi)/1 -> Sum/1
  rcos(phi)/1 -> Sum/2
  qcos(phi)/1 -> Sum1/1
  rsin(phi)/1 -> Sum1/2
  Sum/1 -> tan(theta)(qsin(phi)+rcos(phi))/1, (qsin(phi)+rcos(phi))/cos(theta)/1
  tan(theta)/1 -> tan(theta)(qsin(phi)+rcos(phi))/2
  cos(theta)/1 -> (qsin(phi)+rcos(phi))/cos(theta)/2
  Demux/1 -> Sum2/1
  tan(theta)(qsin(phi)+rcos(phi))/1 -> Sum2/2
  Sum2/1 -> Mux/1
  Sum1/1 -> Mux/2
  (qsin(phi)+rcos(phi))/cos(theta)/1 -> Mux/3
  Mux/1 -> Euler Angles Integrator/1
  Demux2/2 -> pi Bound1/1
  Demux2/1 -> pi Bound/1
  Demux2/3 -> 2pi Bound/1
  pi Bound1/1 -> Mux1/2
  pi Bound/1 -> Mux1/1
  2pi Bound/1 -> Mux1/3
  Euler Angles Integrator/1 -> Demux2/1, Demux1/1
  Mux1/1 -> Euler/1

== system tp333079/Equations of Motion/Body-Frame EOM/Kinematics (Quaternions) ==
  note: Output
  note: Kinematic Equation
  note: Sources
  note: Assemble kinematic transformation matrix
  Rates : Inport  Port=1  PortDimensions=[3 1]  SampleTime=-1  DataType=auto
      settings: SignalType=auto
  RST : Inport  Port=2  PortDimensions=1  SampleTime=-1  DataType=auto
      settings: SignalType=auto
  1/2 : Gain  Gain=0.5  Multiplication=Element-wise(K.*u)  SaturateOnIntegerOverflow=on
  Change Sign : Gain  Gain=-1  Multiplication=Element-wise(K.*u)  SaturateOnIntegerOverflow=on
  Demux : Demux  Outputs=3  BusSelectionMode=off
  Demux1 : Demux  Outputs=3  BusSelectionMode=off
  Kinematic Matrix : simulink3/Signals & Systems/Matrix Concatenation  numInports=4  catMethod=Horizontal
  Kinematic Matrix Col{1..4} (4 alike) : simulink3/Signals & Systems/Matrix Concatenation  numInports=4  catMethod=Vertical
  Km*e : Product  Inputs=2  Multiplication=Matrix(*)  SaturateOnIntegerOverflow=on
  Normalization : Subsystem  Orientation=left  SimViewingDevice=off
      settings: Permissions=ReadWrite  RTWFcnNameOpts=Auto  RTWFileNameOpts=Auto
      mask Type: Vector normalization
      mask Description: Normalize a vector, e = v/|v|
  Quaternion Integrator : Integrator  ExternalReset=rising  InitialConditionSource=internal  InitialCondition=QuaternionsIni  LimitOutput=off  UpperSaturationLimit=inf  LowerSaturationLimit=-inf  ShowSaturationPort=off  ShowStatePort=off  AbsoluteTolerance=auto
  Zero : Constant  Value=0
  Quaternions : Outport  Port=1
  wires:
  Zero/1 -> Kinematic Matrix Col4/4, Kinematic Matrix Col3/3, Kinematic Matrix Col2/2, Kinematic Matrix Col1/1
  Demux1/3 -> Kinematic Matrix Col2/3, Kinematic Matrix Col4/1
  Demux1/2 -> Kinematic Matrix Col4/2, Kinematic Matrix Col3/1
  Demux1/1 -> Kinematic Matrix Col3/4, Kinematic Matrix Col2/1
  Normalization/1(VecOut) -> Km*e/2
  RST/1 -> Quaternion Integrator/2
  Quaternion Integrator/1 -> Quaternions/1, Normalization/1(VecIn)
  1/2/1 -> Quaternion Integrator/1
  Km*e/1 -> 1/2/1
  Kinematic Matrix/1 -> Km*e/1
  Kinematic Matrix Col4/1 -> Kinematic Matrix/4
  Kinematic Matrix Col3/1 -> Kinematic Matrix/3
  Kinematic Matrix Col2/1 -> Kinematic Matrix/2
  Kinematic Matrix Col1/1 -> Kinematic Matrix/1
  Demux/2 -> Kinematic Matrix Col2/4, Kinematic Matrix Col1/3
  Demux/3 -> Kinematic Matrix Col3/2, Kinematic Matrix Col1/4
  Demux/1 -> Kinematic Matrix Col4/3, Kinematic Matrix Col1/2
  Change Sign/1 -> Demux1/1
  Rates/1 -> Change Sign/1, Demux/1

== system tp333079/Equations of Motion/Body-Frame EOM/Moments ==
  note: Output
  note: Moment equation
  note: Get angular accelerations
  note: Sources
  Inertia : Inport  Port=1  PortDimensions=[4 1]  SampleTime=-1  DataType=auto
      settings: SignalType=auto
  Moments : Inport  Port=2  PortDimensions=[3 1]  SampleTime=-1  DataType=auto
      settings: SignalType=auto
  RST : Inport  Port=3  PortDimensions=1  SampleTime=-1  DataType=auto
      settings: SignalType=auto
  (c1r+c2p)q : Product  Inputs=2  Multiplication=Element-wise(.*)  SaturateOnIntegerOverflow=on
  (c8p-c2r)q : Product  Inputs=2  Multiplication=Element-wise(.*)  SaturateOnIntegerOverflow=on
  Demux1 : Demux  Outputs=9  BusSelectionMode=off
  Demux2 : Demux  Outputs=3  BusSelectionMode=off
  Demux4 : Demux  Outputs=3  BusSelectionMode=off
  Inertia Coefficients : aerosimlib/Inertia/Inertia Coefficients
  Mux : Mux  Inputs=3
  Sum : Sum  Inputs=|++  SaturateOnIntegerOverflow=on
  Sum1 : Sum  Inputs=+++  SaturateOnIntegerOverflow=on
  Sum2 : Sum  Inputs=|+-  SaturateOnIntegerOverflow=on
  Sum3 : Sum  Inputs=+-+  SaturateOnIntegerOverflow=on
  Sum4 : Sum  Inputs=|+-  SaturateOnIntegerOverflow=on
  Sum5 : Sum  Inputs=+++  SaturateOnIntegerOverflow=on
  Velocity Integrator : Integrator  ExternalReset=rising  InitialConditionSource=internal  InitialCondition=RatesIni  LimitOutput=off  UpperSaturationLimit=inf  LowerSaturationLimit=-inf  ShowSaturationPort=off  ShowStatePort=off  AbsoluteTolerance=auto
  c1r : Product  Inputs=2  Multiplication=Element-wise(.*)  SaturateOnIntegerOverflow=on
  c2p : Product  Inputs=2  Multiplication=Element-wise(.*)  SaturateOnIntegerOverflow=on
  c2r : Product  Inputs=2  Multiplication=Element-wise(.*)  SaturateOnIntegerOverflow=on
  c3L : Product  Inputs=2  Multiplication=Element-wise(.*)  SaturateOnIntegerOverflow=on
  c4L : Product  Inputs=2  Multiplication=Element-wise(.*)  SaturateOnIntegerOverflow=on
  c4N : Product  Inputs=2  Multiplication=Element-wise(.*)  SaturateOnIntegerOverflow=on
  c5pr : Product  Inputs=3  Multiplication=Element-wise(.*)  SaturateOnIntegerOverflow=on
  c6(p^2-r^2) : Product  Inputs=2  Multiplication=Element-wise(.*)  SaturateOnIntegerOverflow=on
  c7M : Product  Inputs=2  Multiplication=Element-wise(.*)  SaturateOnIntegerOverflow=on
  c8p : Product  Inputs=2  Multiplication=Element-wise(.*)  SaturateOnIntegerOverflow=on
  c9N : Product  Inputs=2  Multiplication=Element-wise(.*)  SaturateOnIntegerOverflow=on
  p^2 : Math  Operator=square  OutputSignalType=auto
  r^2 : Math  Operator=square  OutputSignalType=auto
  Angular Rates : Outport  Port=1
  Angular Acc : Outport  Port=2
  wires:
  Demux4/2 -> (c8p-c2r)q/2, (c1r+c2p)q/2
  Demux4/3 -> c5pr/3, r^2/1, c2r/2, c1r/2
  Demux1/3 -> c3L/1
  Demux1/2 -> c2r/1, c2p/1
  Velocity Integrator/1 -> Angular Rates/1, Demux4/1
  RST/1 -> Velocity Integrator/2
  Mux/1 -> Velocity Integrator/1, Angular Acc/1
  Sum5/1 -> Mux/3
  c9N/1 -> Sum5/3
  c4L/1 -> Sum5/2
  (c8p-c2r)q/1 -> Sum5/1
  Demux1/9 -> c9N/1
  Demux1/4 -> c4N/1, c4L/1
  Sum4/1 -> (c8p-c2r)q/1
  c2r/1 -> Sum4/2
  c8p/1 -> Sum4/1
  Demux4/1 -> p^2/1, c8p/2, c5pr/2, c2p/2
  Demux1/8 -> c8p/1
  Sum3/1 -> Mux/2
  c7M/1 -> Sum3/3
  c6(p^2-r^2)/1 -> Sum3/2
  c5pr/1 -> Sum3/1
  Demux1/7 -> c7M/1
  Sum2/1 -> c6(p^2-r^2)/2
  Demux1/6 -> c6(p^2-r^2)/1
  r^2/1 -> Sum2/2
  p^2/1 -> Sum2/1
  Demux1/5 -> c5pr/1
  Sum1/1 -> Mux/1
  c4N/1 -> Sum1/3
  c3L/1 -> Sum1/2
  (c1r+c2p)q/1 -> Sum1/1
  Sum/1 -> (c1r+c2p)q/1
  c2p/1 -> Sum/2
  c1r/1 -> Sum/1
  Demux1/1 -> c1r/1
  Moments/1 -> Demux2/1
  Demux2/2 -> c7M/2
  Demux2/3 -> c9N/2, c4N/2
  Demux2/1 -> c4L/2, c3L/2
  Inertia Coefficients/1 -> Demux1/1
  Inertia/1 -> Inertia Coefficients/1

== system tp333079/Equations of Motion/Body-Frame EOM/Navigation ==
  note: Navigation equation
  note: Position derivatives
  note: Sources
  Velocities : Inport  Port=1  PortDimensions=[3 1]  SampleTime=-1  DataType=auto
      settings: SignalType=auto
  DCM : Inport  Port=2  PortDimensions=[3 3]  SampleTime=-1  DataType=auto
      settings: SignalType=auto
  Rmeridian : Inport  Port=3  PortDimensions=1  SampleTime=-1  DataType=auto
      settings: SignalType=auto
  Rnormal : Inport  Port=4  PortDimensions=1  SampleTime=-1  DataType=auto
      settings: SignalType=auto
  AConGnd : Inport  Port=5  PortDimensions=1  SampleTime=-1  DataType=auto
      settings: SignalType=auto
  RST : Inport  Port=6  PortDimensions=1  SampleTime=-1  DataType=auto
      settings: SignalType=auto
  Altitude Switch : Switch  Threshold=1
  ChSign : Gain  Gain=-1  Multiplication=Element-wise(K.*u)  SaturateOnIntegerOverflow=on
  DCM' : Math  Operator=transpose  OutputSignalType=auto
  Demux1 : Demux  Outputs=3  BusSelectionMode=off
  Demux3 : Demux  Outputs=3  BusSelectionMode=off
  Latitude Bound : Subsystem  SimViewingDevice=off
      settings: Permissions=ReadWrite  RTWFcnNameOpts=Auto  RTWFileNameOpts=Auto
      mask Type: Latitude bound
      mask Description: Bounds the latitude to [-pi/2, pi/2]. When the lower bound is exceeded the latitude is increasing again; when the upper bound is exceeded the latitude is decreasing.
  Longitude Bound : Subsystem  SimViewingDevice=off
      settings: Permissions=ReadWrite  RTWFcnNameOpts=Auto  RTWFileNameOpts=Auto
      mask Type: Longitude bound
      mask Description: Bounds the longitude to [-pi, pi]. When -pi bound is exceeded the longitude wraps back to pi; when the pi bound is exceeded the longitude wraps back to -pi.
  Mux : Mux  Inputs=3
  Mux1 : Mux  Inputs=3
  Position Integrator : Integrator  ExternalReset=rising  InitialConditionSource=internal  InitialCondition=PositionIni  LimitOutput=off  UpperSaturationLimit=inf  LowerSaturationLimit=-inf  ShowSaturationPort=off  ShowStatePort=off  AbsoluteTolerance=auto
  Product : Product  Inputs=2  Multiplication=Matrix(*)  SaturateOnIntegerOverflow=on
  Sum : Sum  Inputs=|++  SaturateOnIntegerOverflow=on
  Sum1 : Sum  Inputs=|++  SaturateOnIntegerOverflow=on
  Ve/(Rn+h)cos(phi) : Product  Inputs=*//  Multiplication=Element-wise(.*)  SaturateOnIntegerOverflow=on
  Vn/(Rm+h) : Product  Inputs=*/  Multiplication=Element-wise(.*)  SaturateOnIntegerOverflow=on
  Zero : Constant  Value=0
  cos(phi) : Trigonometry  Operator=cos  OutputSignalType=auto
  Position : Outport  Port=1
  Gndspd : Outport  Port=2
  wires:
  Latitude Bound/1(Out) -> Mux1/1, cos(phi)/1
  Mux1/1 -> Position/1
  Longitude Bound/1(Out) -> Mux1/2
  Demux3/1 -> Latitude Bound/1(In)
  Demux3/2 -> Longitude Bound/1(In)
  Demux3/3 -> Mux1/3, Sum1/2, Sum/2
  cos(phi)/1 -> Ve/(Rn+h)cos(phi)/3
  Position Integrator/1 -> Demux3/1
  RST/1 -> Position Integrator/2
  Mux/1 -> Position Integrator/1
  Altitude Switch/1 -> Mux/3
  ChSign/1 -> Altitude Switch/3
  Zero/1 -> Altitude Switch/1
  AConGnd/1 -> Altitude Switch/2
  DCM'/1 -> Product/1
  DCM/1 -> DCM'/1
  Ve/(Rn+h)cos(phi)/1 -> Mux/2
  Sum1/1 -> Ve/(Rn+h)cos(phi)/2
  Vn/(Rm+h)/1 -> Mux/1
  Sum/1 -> Vn/(Rm+h)/2
  Rnormal/1 -> Sum1/1
  Rmeridian/1 -> Sum/1
  Product/1 -> Gndspd/1, Demux1/1
  Demux1/2 -> Ve/(Rn+h)cos(phi)/1
  Demux1/3 -> ChSign/1
  Demux1/1 -> Vn/(Rm+h)/1
  Velocities/1 -> Product/2

== system tp333079/Equations of Motion/Geodetic-Frame EOM/Angular Rate ==
  Inertia : Inport  Port=1  PortDimensions=[4 1]  SampleTime=-1  DataType=auto
      settings: SignalType=auto
  Moments : Inport  Port=2  PortDimensions=[3 1]  SampleTime=-1  DataType=auto
      settings: SignalType=auto
  Pos : Inport  Port=3  PortDimensions=[3 1]  SampleTime=-1  DataType=auto
      settings: SignalType=auto
  dPosdt : Inport  Port=4  PortDimensions=[3 1]  SampleTime=-1  DataType=auto
      settings: SignalType=auto
  DCM : Inport  Port=5  PortDimensions=[3 3]  SampleTime=-1  DataType=auto
      settings: SignalType=auto
  RST : Inport  Port=6  PortDimensions=1  SampleTime=-1  DataType=auto
      settings: SignalType=auto
  ChSign : Gain  Gain=-1  Multiplication=Element-wise(K.*u)  SaturateOnIntegerOverflow=on
  ChSign1 : Gain  Gain=-1  Multiplication=Element-wise(K.*u)  SaturateOnIntegerOverflow=on
  Demux1 : Demux  Outputs=3  BusSelectionMode=off
  Demux3 : Demux  Outputs=3  BusSelectionMode=off
  Earth Rot Rate : Constant  Value=7.292115e-5
  Matrix Concatenation : simulink3/Signals & Systems/Matrix Concatenation  numInports=3  catMethod=Vertical
  Moment Eq : aerosimlib/Equations of Motion/Body-Frame EOM/Moments  RatesIni=RatesIni
  Product : Product  Inputs=2  Multiplication=Matrix(*)  SaturateOnIntegerOverflow=on
  Product1 : Product  Inputs=2  Multiplication=Element-wise(.*)  SaturateOnIntegerOverflow=on
  Product2 : Product  Inputs=2  Multiplication=Element-wise(.*)  SaturateOnIntegerOverflow=on
  Sum1 : Sum  Inputs=|++  SaturateOnIntegerOverflow=on
  Sum2 : Sum  Inputs=|+-  SaturateOnIntegerOverflow=on
  Terminator : Terminator
  Terminator1 : Terminator
  Terminator2 : Terminator
  Trigonometric Function : Trigonometry  Operator=sin  OutputSignalType=auto
  Trigonometric Function1 : Trigonometry  Operator=cos  OutputSignalType=auto
  Angular Rate : Outport  Port=1
  Angular Acc : Outport  Port=2
  wires:
  Inertia/1 -> Moment Eq/1
  Moments/1 -> Moment Eq/2
  RST/1 -> Moment Eq/3
  Pos/1 -> Demux3/1
  dPosdt/1 -> Demux1/1
  Earth Rot Rate/1 -> Sum1/2
  Demux1/2 -> Sum1/1
  Demux3/1 -> Trigonometric Function1/1, Trigonometric Function/1
  Demux3/2 -> Terminator/1
  Demux3/3 -> Terminator1/1
  Demux1/3 -> Terminator2/1
  Sum1/1 -> Product1/1, Product2/1
  Trigonometric Function1/1 -> Product1/2
  Product1/1 -> Matrix Concatenation/1
  Trigonometric Function/1 -> Product2/2
  Product2/1 -> ChSign/1
  Demux1/1 -> ChSign1/1
  ChSign1/1 -> Matrix Concatenation/2
  ChSign/1 -> Matrix Concatenation/3
  Matrix Concatenation/1 -> Product/2
  DCM/1 -> Product/1
  Moment Eq/1 -> Sum2/1
  Product/1 -> Sum2/2
  Sum2/1 -> Angular Rate/1
  Moment Eq/2 -> Angular Acc/1
